simulink model "lift_flowchart"  (R2020a)
settings: Solver=VariableStepAuto  StartTime=0.0  StopTime=10.0  RelTol=1e-3
settings Model: Creator=kiran  LastModifiedBy=kiran

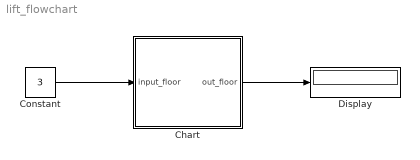
== system lift_flowchart ==
  Chart : Stateflow chart  TreatAsAtomicUnit=on
  Constant : Constant  Value=3
  Display : Display
  wires:
  Constant/1 -> Chart/1(input_floor)
  Chart/1(out_floor) -> Display/1

== stateflow chart lift_flowchart/Chart ==
  (default) -> (junction 9)
  (junction 9) -> (junction 17) [order 1] : [current_floor<input_floor]
  (junction 9) -> (junction 5) [order 2]
  (junction 17) -> (junction 19) : {current_floor=current_floor+1;}
  (junction 5) -> (junction 23) [order 1] : [current_floor>input_floor]
  (junction 5) -> (junction 18) [order 2]
  (junction 23) -> (junction 21) : {current_floor=current_floor-1;}
  (junction 18) -> (junction 24) [order 1] : [current_floor==input_floor]
  (junction 18) -> (junction 22) [order 2] : {current_floor=0;}
  (junction 24) -> (junction 25) : {current_floor=input_floor;}
  (junction 25) -> (junction 22)
  (junction 21) -> (junction 25)
  (junction 19) -> (junction 21)
  (junction 22) -> (junction 20) : {out_floor=current_floor}
  data: input_floor input; out_floor output; current_floor local =0
